simulink model "plotting_with_filter"  (R2018b)
settings: Solver=VariableStepAuto  StartTime=0.0  StopTime=1000  RelTol=1e-3
libraries: simulink_extras x1
settings Model: Creator=Tejas Rajopadhye  LastModifiedBy=Tejas Rajopadhye

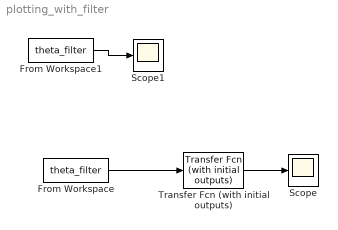
== system plotting_with_filter ==
  From Workspace : FromWorkspace  VariableName=theta_filter  SampleTime=0
  From Workspace1 : FromWorkspace  VariableName=theta_filter  SampleTime=0
  Scope : Scope
  Scope1 : Scope
  Transfer Fcn (with initial outputs) : simulink_extras/Additional Linear/Transfer Fcn (with initial outputs)  N=[0.005]  D="[1  1]"  Y0=0  U0=0
  wires:
  From Workspace/1 -> Transfer Fcn (with initial outputs)/1
  Transfer Fcn (with initial outputs)/1 -> Scope/1
  From Workspace1/1 -> Scope1/1
